simulink model "DM_2"  (Simulink 8.1)
settings: Solver=ode45  StartTime=0.0  StopTime=10.0  RelTol=1e-3
libraries: xbsIndex_r4 x16
settings Model: Creator=SAYANTAN  LastModifiedBy=SAYANTAN
settings DataIOCC: SignalLoggingSaveFormat=Dataset
settings OptimizationCC: ExpressionDepthLimit=128
settings DebuggingCC: FcnCallInpInsideContextMsg=EnableAllAsError
settings GRTTargetCC: CombineOutputUpdateFcns=on  GRTInterface=off

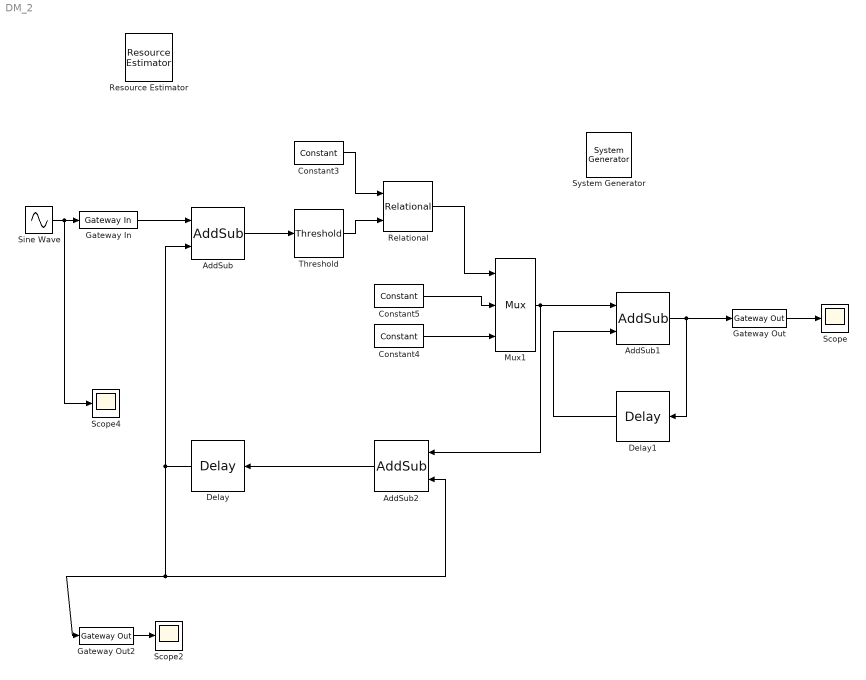
== system DM_2 ==
  " System Generator" : xbsIndex_r4/ System Generator  Tag=genX  xilinxfamily=kintex7  part=xc7k325t  speed=-3  package=fbg676  synthesis_tool=XST  clock_wrapper=Clock Enables  directory=./netlist  proj_type=Project Navigator  Synth_file=XST Defaults  Impl_file=ISE Defaults  testbench=off  simulink_period=0.005  sysclk_period=10  dcm_input_clock_period=10  incr_netlist=off  trim_vbits=Everywhere in SubSystem  dbl_ovrd=According to Block Masks  core_generation=According to Block Masks  run_coregen=off  deprecated_control=off  eval_field=0  block_type=sysgen
  AddSub : xbsIndex_r4/AddSub  mode=Subtraction  use_carryin=off  use_carryout=off  en=off  latency=0  precision=User Defined  arith_type="Signed  (2's comp)"  n_bits=22  bin_pt=14  quantization=Truncate  overflow=Wrap  dbl_ovrd=off  use_behavioral_HDL=off  hw_selection=Fabric  pipelined=off  block_type=addsub
      settings: xl_area=[11 0 0 22 0 0 0]
  AddSub1 : xbsIndex_r4/AddSub  mode=Addition  use_carryin=off  use_carryout=off  en=off  latency=0  precision=User Defined  arith_type="Signed  (2's comp)"  n_bits=22  bin_pt=14  quantization=Truncate  overflow=Wrap  dbl_ovrd=off  use_behavioral_HDL=off  hw_selection=Fabric  pipelined=off  block_type=addsub
      settings: xl_area=[11 0 0 22 0 0 0]
  AddSub2 : xbsIndex_r4/AddSub  mode=Addition  use_carryin=off  use_carryout=off  en=off  latency=0  precision=User Defined  arith_type="Signed  (2's comp)"  n_bits=22  bin_pt=14  quantization=Truncate  overflow=Wrap  dbl_ovrd=off  use_behavioral_HDL=off  hw_selection=Fabric  pipelined=off  block_type=addsub
      settings: xl_area=[11 0 0 22 0 0 0]
  Constant3 : xbsIndex_r4/Constant  const=-1  gui_display_data_type=Fixed-point  arith_type=Signed (2's comp)  n_bits=16  bin_pt=14  preci_type=Single  exp_width=8  frac_width=24  explicit_period=off  period=1  equ=P=C  opselect=C  inp2=PCIN>>17  opr=+  inp1=P  carry=CIN  dbl_ovrd=off  block_type=constant
  Constant4 : xbsIndex_r4/Constant  const=-0.1256  gui_display_data_type=Fixed-point  arith_type=Signed (2's comp)  n_bits=16  bin_pt=14  preci_type=Single  exp_width=8  frac_width=24  explicit_period=off  period=1  equ=P=C  opselect=C  inp2=PCIN>>17  opr=+  inp1=P  carry=CIN  dbl_ovrd=off  block_type=constant
  Constant5 : xbsIndex_r4/Constant  const=0.1256  gui_display_data_type=Fixed-point  arith_type=Signed (2's comp)  n_bits=16  bin_pt=14  preci_type=Single  exp_width=8  frac_width=24  explicit_period=off  period=1  equ=P=C  opselect=C  inp2=PCIN>>17  opr=+  inp1=P  carry=CIN  dbl_ovrd=off  block_type=constant
  Delay : xbsIndex_r4/Delay  rst=off  infoeditControl=Selection of Reset will increase slice count due to use of real FFs and instead of SRLs  en=off  latency=1  dbl_ovrd=off  reg_retiming=off  block_type=delay
      settings: xl_area=[11 22 0 0 0 0 0]
  Delay1 : xbsIndex_r4/Delay  rst=off  infoeditControl=Selection of Reset will increase slice count due to use of real FFs and instead of SRLs  en=off  latency=1  dbl_ovrd=off  reg_retiming=off  block_type=delay
      settings: xl_area=[11 22 0 0 0 0 0]
  Gateway In : xbsIndex_r4/Gateway In  gui_display_data_type=Fixed-point  arith_type="Signed  (2's comp)"  n_bits=22  bin_pt=14  preci_type=Single  exp_width=8  frac_width=24  quantization="Round  (unbiased: +/- Inf)"  overflow=Saturate  period=0.005  dbl_ovrd=off  timing_constraint=None  locs_specified=off  LOCs={}  UseAsADC=off  ADCChannel='1'  inherit_from_input=off  hdl_port=on  block_type=gatewayin
      settings: xl_area=[0 0 0 0 22 0 0]
  Gateway Out : xbsIndex_r4/Gateway Out  inherit_from_input=off  hdl_port=on  timing_constraint=None  locs_specified=off  LOCs={}  UseAsDAC=off  DACChannel='1'  block_type=gatewayout
      settings: xl_area=[0 0 0 0 22 0 0]
  Gateway Out2 : xbsIndex_r4/Gateway Out  inherit_from_input=off  hdl_port=on  timing_constraint=None  locs_specified=off  LOCs={}  UseAsDAC=off  DACChannel='1'  block_type=gatewayout
      settings: xl_area=[0 0 0 0 22 0 0]
  Mux1 : xbsIndex_r4/Mux  inputs=2  en=off  latency=0  precision=Full  arith_type=Unsigned  n_bits=16  bin_pt=14  quantization=Truncate  overflow=Wrap  dbl_ovrd=off  block_type=mux
      settings: xl_area=[8 0 0 16 0 0 0]
  Relational : xbsIndex_r4/Relational  mode=a=b  en=off  latency=0  dbl_ovrd=off  block_type=relational
      settings: xl_area=[4 0 0 8 0 0 0]
  Resource Estimator : xbsIndex_r4/Resource Estimator  Tag=resEstTag  Slices=0  FFs=0  BRAMs=0  LUTs=0  IOBs=0  EBMs=0  TBUFs=0  xl_use_estimator_area=off  est_options=Estimate  xl_estimator_area=[67 44 0 90 104 0 0]  block_type=resource_estimator
      settings: AttributesFormatString=Resource\nEstimator
  Scope : Scope
  Scope2 : Scope
      settings: SaveName=ScopeData2
  Scope4 : Scope
      settings: SaveName=ScopeData4
  Sine Wave : Sin  Amplitude=2  Frequency=2  SampleTime=0
  Threshold : xbsIndex_r4/Threshold  en=off  latency=0  dbl_ovrd=off  block_type=sgn
      settings: infoedit="Presents -1 as output if input is negative; otherwise presents 1.  Output is a two bit signed number."  xl_area=[0 0 0 0 0 0 0]
  wires:
  AddSub/1 -> Threshold/1
  Threshold/1 -> Relational/2
  Constant3/1 -> Relational/1
  Constant4/1 -> Mux1/3
  Constant5/1 -> Mux1/2
  Mux1/1 -> AddSub1/1, AddSub2/1
  Delay/1 -> AddSub2/2, Gateway Out2/1, AddSub/2
  Gateway In/1 -> AddSub/1
  Sine Wave/1 -> Scope4/1, Gateway In/1
  Delay1/1 -> AddSub1/2
  AddSub1/1 -> Delay1/1, Gateway Out/1
  Gateway Out/1 -> Scope/1
  Gateway Out2/1 -> Scope2/1
  Relational/1 -> Mux1/1
  AddSub2/1 -> Delay/1
